simulink model "ex1_3"  (R2020a)
settings: Solver=ode45  StartTime=0.0  StopTime=10.0  MaxStep=1e-2  RelTol=1e-3
settings Model: Creator=반달  LastModifiedBy=반달

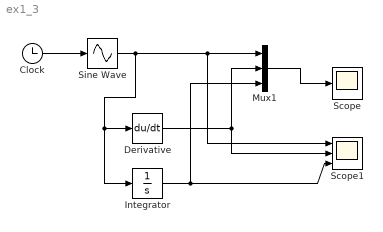
== system ex1_3 ==
  Clock : Clock
  Derivative : Derivative
  Integrator : Integrator
  Mux1 : Mux  Inputs=3
  Scope : Scope
  Scope1 : Scope  NumInputPorts=3
  Sine Wave : Sin  TimeSource=Use external signal  Frequency=2*pi*0.25  SampleTime=0
  wires:
  Clock/1 -> Sine Wave/1
  Sine Wave/1 -> Integrator/1, Derivative/1, Scope1/1, Mux1/1
  Derivative/1 -> Scope1/2, Mux1/2
  Mux1/1 -> Scope/1
  Integrator/1 -> Mux1/3, Scope1/3
